simulink model "E2s"  (R2014a)
settings: Solver=ode45  StartTime=0.0  StopTime=10  RelTol=1e-20
values from neighbouring files (symbols this model uses):
  A = 9    [E2.m]
libraries: cstblocks x2, simulink x2
settings Model: Creator=Davide  LastModifiedBy=Davide

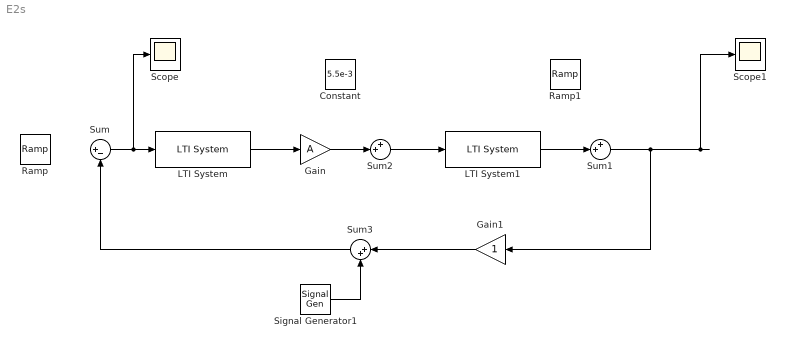
== system E2s ==
  Constant : Constant  Value=5.5e-3
  Gain : Gain  Gain=A
  Gain1 : Gain
  LTI System : cstblocks/LTI System  sys=C  IC=[]
  LTI System1 : cstblocks/LTI System  sys=Gp  IC=[]
  Ramp : simulink/Sources/Ramp  slope=1  start=0  X0=0
  Ramp1 : simulink/Sources/Ramp  slope=5.5e-3  start=0  X0=0
  Scope : Scope
  Scope1 : Scope
  Signal Generator1 : SignalGenerator  Amplitude=1e-3  Frequency=30  Units=rad/sec
  Sum : Sum  Inputs=|+-
  Sum1 : Sum  Inputs=++|
  Sum2 : Sum  Inputs=++|
  Sum3 : Sum  Inputs=|++
  wires:
  Sum/1 -> Scope/1, LTI System/1
  LTI System/1 -> Gain/1
  Sum1/1 -> Gain1/1, Scope1/1
  Gain/1 -> Sum2/2
  LTI System1/1 -> Sum1/2
  Sum2/1 -> LTI System1/1
  Gain1/1 -> Sum3/1
  Sum3/1 -> Sum/2
  Signal Generator1/1 -> Sum3/2
